simulink model "p54_pendulum_sim"  (R2023a)
settings: Solver=VariableStepAuto  StartTime=0.0  StopTime=Tf  MaxStep=MaxStep  RelTol=RelTol
values from neighbouring files (symbols this model uses):
  b = 0.05    [p54_pendulum.m]    (also in p54_pendulum_runme.m)
  C_star = M*g*l*sin(theta_star)    [p54_pendulum.m]    (also in p54_pendulum_runme.m)
  g = 9.81    [p54_pendulum.m]    (also in p54_pendulum_runme.m)
  l = 0.3    [p54_pendulum.m]    (also in p54_pendulum_runme.m)
  M = 0.5    [p54_pendulum.m]    (also in p54_pendulum_runme.m)
  theta_star = pi/3    (= 1.0471975512)    [p54_pendulum.m]    (also in p54_pendulum_runme.m)
  x0 = [pi/3; 0]    [p54_pendulum.m]    (also in p54_pendulum_runme.m)
undefined symbols (not defined in the file or in its folder): den, num
settings Model: Creator=alessandro  LastModifiedBy=admin
settings OptimizationCC: ReuseModelBlockBuffer=off

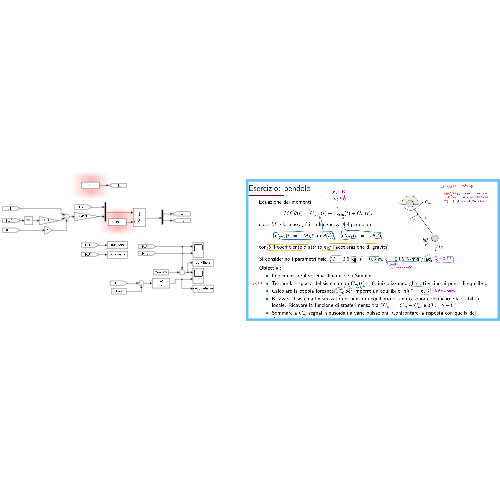
[thumbnail: Simulink's stored preview of the top-level diagram]
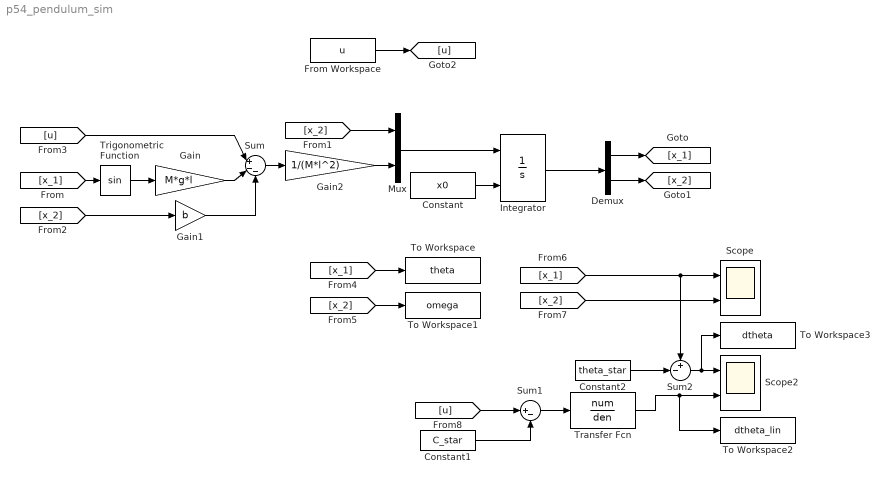
== system p54_pendulum_sim ==
  Constant : Constant  Value=x0
  Constant1 : Constant  Value=C_star
  Constant2 : Constant  Value=theta_star
  Demux : Demux  Outputs=2
  From Workspace : FromWorkspace  VariableName=u
  Gain : Gain  Gain=M*g*l
  Gain1 : Gain  Gain=b
  Gain2 : Gain  Gain=1/(M*l^2)
  Integrator : Integrator  InitialConditionSource=external
  Mux : Mux  Inputs=2
  Scope : Scope  NumInputPorts=2
  Scope2 : Scope  NumInputPorts=2
  Sum : Sum  Inputs=|+--
  Sum1 : Sum  Inputs=|+-
  Sum2 : Sum  Inputs=+-|
  To Workspace : ToWorkspace  VariableName=theta  SaveFormat=Timeseries  SampleTime=-1
  To Workspace1 : ToWorkspace  VariableName=omega  SaveFormat=Timeseries  SampleTime=-1
  To Workspace2 : ToWorkspace  VariableName=dtheta_lin  SaveFormat=Timeseries  SampleTime=-1
  To Workspace3 : ToWorkspace  VariableName=dtheta  SaveFormat=Timeseries  SampleTime=-1
  Transfer Fcn : TransferFcn  Numerator=num  Denominator=den
  Trigonometric Function : Trigonometry
  wires:
  Constant/1 -> Integrator/2
  Mux/1 -> Integrator/1
  Integrator/1 -> Demux/1
  Demux/1 -> [x_1]
  Demux/2 -> [x_2]
  [x_2] -> Mux/1
  Sum/1 -> Gain2/1
  [x_1] -> Trigonometric Function/1
  [x_2] -> Gain1/1
  Gain1/1 -> Sum/3
  Gain2/1 -> Mux/2
  [u] -> Sum/1
  Trigonometric Function/1 -> Gain/1
  From Workspace/1 -> [u]
  [x_1] -> To Workspace/1
  [x_2] -> To Workspace1/1
  [x_1] -> Sum2/1, Scope/1
  [x_2] -> Scope/2
  Gain/1 -> Sum/2
  Sum1/1 -> Transfer Fcn/1
  Transfer Fcn/1 -> To Workspace2/1, Scope2/2
  [u] -> Sum1/1
  Constant1/1 -> Sum1/2
  Sum2/1 -> To Workspace3/1, Scope2/1
  Constant2/1 -> Sum2/2
